simulink model "OutputToStimulatorAMS3800"  (R2016b)
settings: Solver=FixedStepDiscrete  StartTime=0.0  StopTime=inf  FixedStep=sCoreParams.core.stepPeriod  RelTol=1e-3
undefined symbols (not defined in the file or in its folder): sCoreParams, sCoreParams_stimulator_refractoryPeriodSec, sCoreParams_stimulator_startupTimeSec
libraries: xpcparallelportlib x1
Description:
  | This model consists of the simulator configuration and the output to the parallel port.
  | Inputs:
  |   1. isEventDetected: 1 if event was detected 0 if NO event.
  |   2. sendStimPulse: 1 if a stimulus should be sent
  | An example of the usage if this two inputs follows. We could have 2 reason to perform a stimulation (e.g. event detected or sham).
  | In that case input 1 will be 1 only when event is detected while input 2 will be 1 for both stimulations.
  | 
  | Outputs:
  |   1. StimHappening: Indicates that a stimulation pulse was sent through the parallel port to the cerexstim
settings Model: Creator=rzelmann  LastModifiedBy=rzelmann
settings SolverCC: EnableConcurrentExecution=on  AutoInsertRateTranBlk=on
settings DataIOCC: LimitDataPoints=on  SaveFormat=StructureWithTime  SaveOutput=off  SignalLogging=off  SaveTime=off
settings OptimizationCC: BlockReduction=off  DefaultParameterBehavior=Inlined  OptimizeBlockIOStorage=off  BufferReuse=off  GlobalBufferReuse=off  ExpressionFolding=off  LocalBlockOutputs=off  LifeSpan=inf
settings DebuggingCC: AlgebraicLoopMsg=error  SingleTaskRateTransMsg=error  AllowSymbolicDim=off  SFUnexpectedBacktrackingDiag=warning  SFNoUnconditionalDefaultTransitionDiag=warning  SFExecutionAtInitializationDiag=none
settings HardwareCC: ProdBitPerPointer=32  ProdBitPerSizeT=32  ProdBitPerPtrDiffT=32  ProdLargestAtomicFloat=None  ProdWordSize=32  ProdLongLongMode=on  ProdHWDeviceType=Generic->32-bit x86 compatible
settings ModelReferenceCC: ModelReferenceNumInstancesAllowed=Single  ModelReferencePassRootInputsByReference=off
settings RTWCC: SystemTargetFile=slrt.tlc  TemplateMakefile=slrt_default_tmf  Description=Simulink Real-Time  RTWCompilerOptimization=on
settings ConfigComp: CovMetricSettings=dw  CovHtmlReporting=on  CovSaveCumulativeToWorkspaceVar=on  CovSaveSingleToWorkspaceVar=on  CovExternalEMLEnable=off

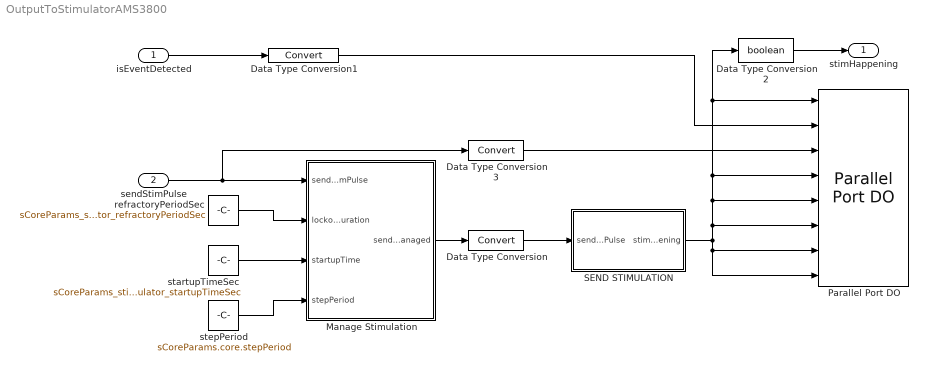
== system OutputToStimulatorAMS3800 ==
  isEventDetected : Inport  OutDataTypeStr=boolean  SampleTime=sCoreParams.core.stepPeriod
  sendStimPulse : Inport  Port=2  OutDataTypeStr=boolean  SampleTime=sCoreParams.core.stepPeriod
  Data Type Conversion : DataTypeConversion
  Data Type Conversion1 : DataTypeConversion
  Data Type Conversion2 : DataTypeConversion  OutDataTypeStr=boolean
  Data Type Conversion3 : DataTypeConversion
  Manage Stimulation : MATLAB Function  TreatAsAtomicUnit=on  SystemSampleTime=sCoreParams.core.stepPeriod
  "Parallel Port DO " : xpcparallelportlib/Digital Output/Parallel Port DO   BaseMask=0x378  BaseString=0x378  Format=8 1-bit Channels  Channels=[1:8]  InitialValues=[0]  FinalActions=[0]  FinalValues=[0]  SampleTime=sCoreParams.core.stepPeriod  Mode=1
  SEND STIMULATION : MATLAB Function  TreatAsAtomicUnit=on
  refractoryPeriodSec : Constant  Value=sCoreParams_stimulator_refractoryPeriodSec
  startupTimeSec : Constant  Value=sCoreParams_stimulator_startupTimeSec
  stepPeriod : Constant  Value=sCoreParams.core.stepPeriod
  stimHappening : Outport  OutDataTypeStr=boolean  SampleTime=sCoreParams.core.stepPeriod
  wires:
  stepPeriod/1 -> Manage Stimulation/4(stepPeriod)
  startupTimeSec/1 -> Manage Stimulation/3(startupTime)
  refractoryPeriodSec/1 -> Manage Stimulation/2(lockoutDuration)
  sendStimPulse/1 -> Data Type Conversion3/1, Manage Stimulation/1(sendStimPulse)
  SEND STIMULATION/1(stimHappening) -> "Parallel Port DO "/6, Data Type Conversion2/1, "Parallel Port DO "/1, "Parallel Port DO "/4, "Parallel Port DO "/5, "Parallel Port DO "/8, "Parallel Port DO "/7
  Manage Stimulation/1(sendStimManaged) -> Data Type Conversion/1
  isEventDetected/1 -> Data Type Conversion1/1
  Data Type Conversion1/1 -> "Parallel Port DO "/2
  Data Type Conversion2/1 -> stimHappening/1
  Data Type Conversion3/1 -> "Parallel Port DO "/3
  Data Type Conversion/1 -> SEND STIMULATION/1(sendStimPulse)

== matlab function OutputToStimulatorAMS3800/SEND STIMULATION ==
  data: sendStimPulse input; stimHappening output
function stimHappening = sendStimToAMS3800(sendStimPulse)
%#codegen

stimHappening = sendStimToAMS3800_EML(sendStimPulse);

== matlab function OutputToStimulatorAMS3800/Manage Stimulation ==
  data: sendStimPulse input; sendStimManaged output; lockoutDuration input; startupTime input; stepPeriod input
function sendStimManaged = ManageStimLockout(sendStimPulse,lockoutDuration,startupTime,stepPeriod)
%#codegen

sendStimManagedB = ManageStimLockout_EML(sendStimPulse,lockoutDuration,startupTime,stepPeriod);
sendStimManaged = double(sendStimManagedB);
